simulink model "URController"  (R2023a)
settings: Solver=ode4  StartTime=0.0  StopTime=3  FixedStep=0.001  RelTol=1e-3  EnableMultiTasking=on
values from neighbouring files (symbols this model uses):
  CYCLE_FREQ = 0.001    [init.m]
  MAX_ACC = 100    [init.m]
  MAX_VEL = 180    [init.m]
libraries: slpidlib x13, forwardkinematics x2, simulink x1
(part 1 of 3)
settings Model: Creator=Steve  LastModifiedBy=Steve
settings SolverCC: AutoInsertRateTranBlk=on
settings DataIOCC: SaveOutput=off  SaveTime=off
settings OptimizationCC: DefaultParameterBehavior=Inlined  InlineInvariantSignals=on  EnhancedBackFolding=on  PassReuseOutputArgsAs=Individual arguments  StateBitsets=on  DataBitsets=on  ZeroExternalMemoryAtStartup=off  ZeroInternalMemoryAtStartup=off  NoFixptDivByZeroProtection=on  LifeSpan=1  OptimizeBlockOrder=speed  DifferentSizesBufferReuse=on  EfficientTunableParamExpr=on
settings DebuggingCC: ParameterTunabilityLossMsg=error  UnderSpecifiedDimensionMsg=warning
settings HardwareCC: ProdBitPerPointer=32  ProdBitPerSizeT=32  ProdBitPerPtrDiffT=32  ProdLargestAtomicFloat=None  ProdIntDivRoundTo=Floor  ProdWordSize=32  ProdHWDeviceType=Generic->Custom
settings SFSimCC: MATLABDynamicMemAlloc=off
settings RTWCC: Description=Embedded Coder  SystemTargetFile=ert.tlc  TLCOptions=-p0  GenCodeOnly=on  PackageGeneratedCodeAndArtifacts=on  TemplateMakefile=ert_default_tmf  GenerateReport=on  RTWVerbose=off  IncludeHyperlinkInReport=on  LaunchReport=on  TargetLang=C++
settings CodeAppCC: ForceParamTrailComments=on  IgnoreCustomStorageClasses=off  OperatorAnnotations=on  SimulinkDataObjDesc=on  SFDataObjDesc=on  CustomSymbolStrGlobalVar=rt$N$M  CustomSymbolStrType=$N$M  CustomSymbolStrFcn=$N$M$F  CustomSymbolStrMacro=$N$M  InsertBlockDesc=on
settings ERTTargetCC: TargetLangStandard=C++11 (ISO)  CodeReplacementLibrary=ISO_C  GenerateSampleERTMain=on  SupportAbsoluteTime=off  CodeInterfacePackaging=C++ class  SupportNonFinite=off  SupportComplex=off  SupportContinuousTime=on  SupportVariableSizeSignals=on  InlinedParameterPlacement=NonHierarchical  RootIOFormat=Structure reference  ERTDataSrcFileTemplate=data_h_template.cgt  ERTCustomFileTemplate=example_file_process.tlc

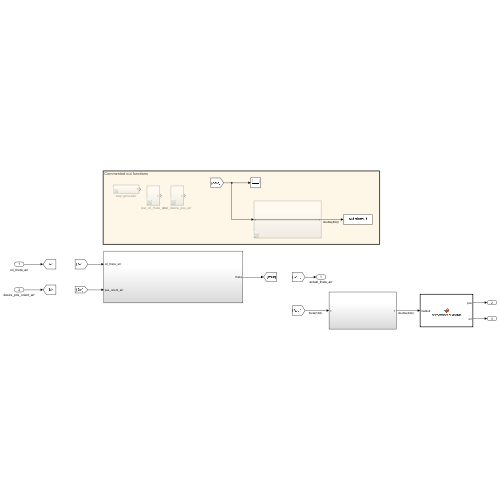
[thumbnail: Simulink's stored preview of the top-level diagram]
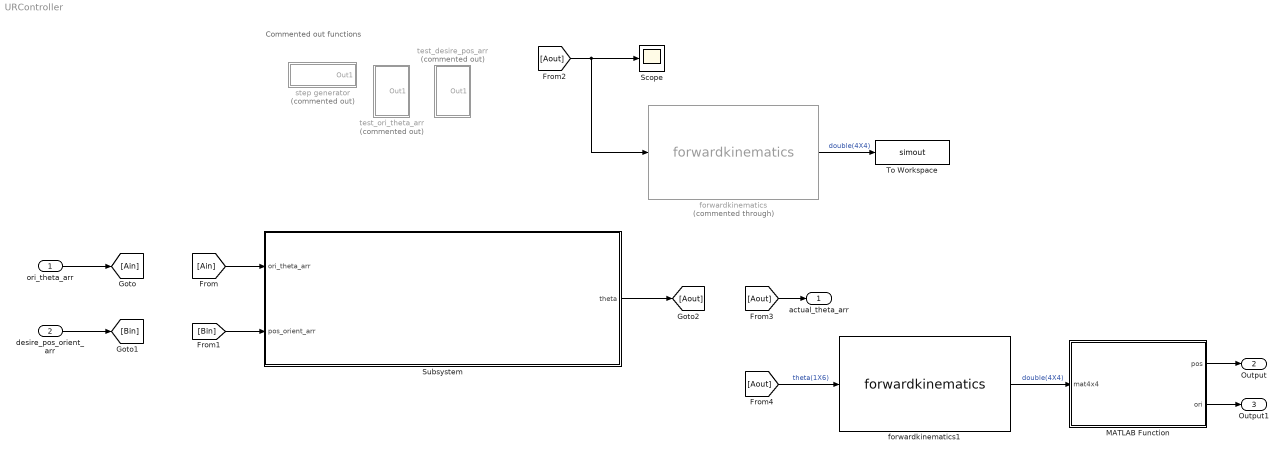
== system URController ==
  note: Commented out functions
  ori_theta_arr : Inport  OutDataTypeStr=double  PortDimensions=6
  desire_pos_orient_arr : Inport  Port=2  OutDataTypeStr=double  PortDimensions=6
  MATLAB Function : MATLAB Function  TreatAsAtomicUnit=on
  Scope : Scope
  Subsystem : Subsystem
  To Workspace : ToWorkspace  VariableName=simout  SaveFormat=Timeseries  SampleTime=-1
  forwardkinematics : forwardkinematics/forwardkinematics  Commented=through  SystemSampleTime=-1  VariantActivationTime=update diagram  Latency=0  AutoFrameSizeCalculation=off
      settings: SourceProductName=My Library
  forwardkinematics1 : forwardkinematics/forwardkinematics  SystemSampleTime=-1  VariantActivationTime=update diagram  Latency=0  AutoFrameSizeCalculation=off
      settings: SourceProductName=My Library
  step generator : Subsystem  Commented=on
  test_desire_pos_arr : Subsystem  Commented=on
  test_ori_theta_arr : Subsystem  Commented=on
  actual_theta_arr : Outport  OutDataTypeStr=double  PortDimensions=6
  Output : Outport  Port=2
  Output1 : Outport  Port=3
  wires:
  [Aout] -> Scope/1, forwardkinematics/1
  forwardkinematics/1 -> To Workspace/1  "double(4X4)"
  [Ain] -> Subsystem/1(ori_theta_arr)
  [Bin] -> Subsystem/2(pos_orient_arr)
  Subsystem/1(theta) -> [Aout]
  [Aout] -> actual_theta_arr/1
  [Aout] -> forwardkinematics1/1  "theta(1X6)"
  ori_theta_arr/1 -> [Ain]
  desire_pos_orient_arr/1 -> [Bin]
  forwardkinematics1/1 -> MATLAB Function/1(mat4x4)  "double(4X4)"
  MATLAB Function/1(pos) -> Output/1
  MATLAB Function/2(ori) -> Output1/1

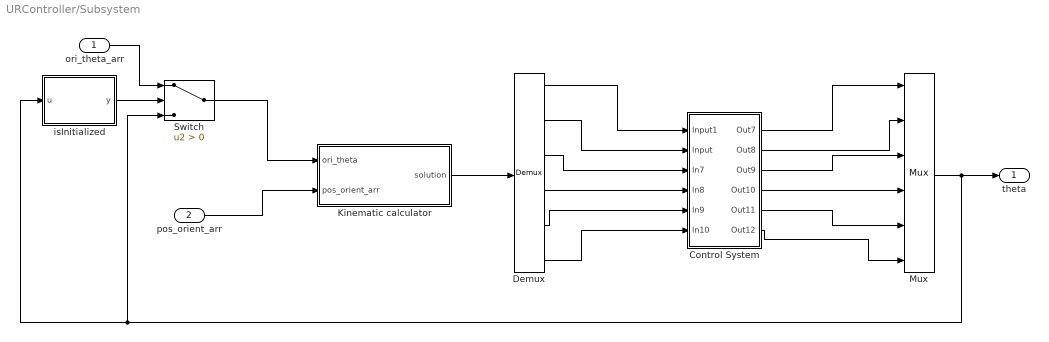
== system URController/Subsystem ==
  ori_theta_arr : Inport
  pos_orient_arr : Inport  Port=2
  Control System : Subsystem
  Demux : Demux  Outputs=6
  Kinematic calculator : Subsystem
  Mux : Mux  Inputs=6
  Switch : Switch  Criteria=u2 > Threshold  SaturateOnIntegerOverflow=off  InputSameDT=off
  isInitialized : MATLAB Function  TreatAsAtomicUnit=on
  theta : Outport
  wires:
  Mux/1 -> theta/1, isInitialized/1(u), Switch/3
  ori_theta_arr/1 -> Switch/1
  Switch/1 -> Kinematic calculator/1(ori_theta)
  Kinematic calculator/1(solution) -> Demux/1
  pos_orient_arr/1 -> Kinematic calculator/2(pos_orient_arr)
  isInitialized/1(y) -> Switch/2
  Demux/1 -> Control System/1(Input1)
  Demux/2 -> Control System/2(Input)
  Demux/3 -> Control System/3(In7)
  Demux/4 -> Control System/4(In8)
  Demux/5 -> Control System/5(In9)
  Demux/6 -> Control System/6(In10)
  Control System/1(Out7) -> Mux/1
  Control System/2(Out8) -> Mux/2
  Control System/3(Out9) -> Mux/3
  Control System/4(Out10) -> Mux/4
  Control System/5(Out11) -> Mux/5
  Control System/6(Out12) -> Mux/6

== system URController/step generator ==
  Clock : Clock
  Constant12 : Constant
  Constant13 : Constant  Value=[1 , 5 , 10 ,15]
  Floor : Rounding
  Selector : Selector  InputPortWidth=4  IndexOptions=Index vector (port)  Indices=[1 3]  OutputSizes=1
  Sum6 : Sum  Inputs=|++
  Out1 : Outport
  wires:
  Constant12/1 -> Sum6/2
  Constant13/1 -> Selector/1
  Selector/1 -> Out1/1
  Sum6/1 -> Floor/1
  Floor/1 -> Selector/2  "alpha"
  Clock/1 -> Sum6/1

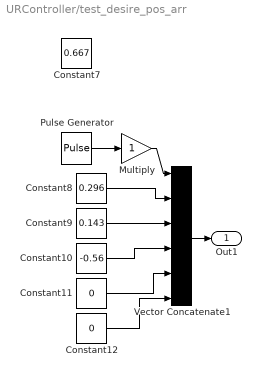
== system URController/test_desire_pos_arr ==
  Constant10 : Constant  Value=-0.56  OutDataTypeStr=double
  Constant11 : Constant  Value=0  OutDataTypeStr=double
  Constant12 : Constant  Value=0  OutDataTypeStr=double
  Constant7 : Constant  Value=0.667  OutDataTypeStr=double
  Constant8 : Constant  Value=0.296  OutDataTypeStr=double
  Constant9 : Constant  Value=0.143  OutDataTypeStr=double
  Multiply : Gain
  Pulse Generator : DiscretePulseGenerator  PulseType=Time based  Amplitude=0.01  Period=1  PulseWidth=20
  Vector Concatenate1 : Concatenate  NumInputs=6
  Out1 : Outport
  wires:
  Vector Concatenate1/1 -> Out1/1
  Constant12/1 -> Vector Concatenate1/6
  Constant11/1 -> Vector Concatenate1/5
  Constant9/1 -> Vector Concatenate1/3
  Constant10/1 -> Vector Concatenate1/4
  Pulse Generator/1 -> Multiply/1
  Constant8/1 -> Vector Concatenate1/2
  Multiply/1 -> Vector Concatenate1/1

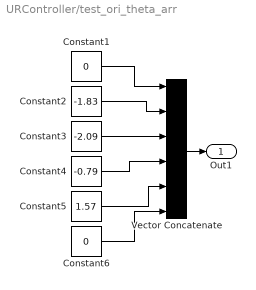
== system URController/test_ori_theta_arr ==
  Constant1 : Constant  Value=0  OutDataTypeStr=double
  Constant2 : Constant  Value=-1.83  OutDataTypeStr=double
  Constant3 : Constant  Value=-2.09  OutDataTypeStr=double
  Constant4 : Constant  Value=-0.79  OutDataTypeStr=double
  Constant5 : Constant  Value=1.57  OutDataTypeStr=double
  Constant6 : Constant  Value=0  OutDataTypeStr=double
  Vector Concatenate : Concatenate  NumInputs=6
  Out1 : Outport
  wires:
  Constant3/1 -> Vector Concatenate/3
  Constant4/1 -> Vector Concatenate/4
  Constant2/1 -> Vector Concatenate/2
  Constant1/1 -> Vector Concatenate/1
  Constant6/1 -> Vector Concatenate/6
  Constant5/1 -> Vector Concatenate/5
  Vector Concatenate/1 -> Out1/1

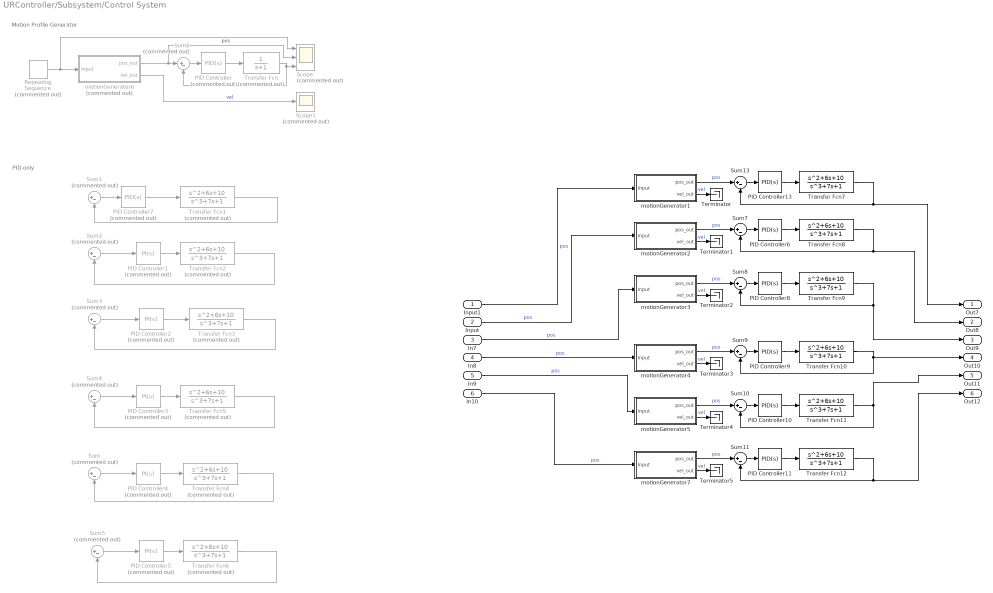
== system URController/Subsystem/Control System ==
  note: PID only
  note: Motion Profile Generator
  Input1 : Inport
  Input : Inport  Port=2
  In7 : Inport  Port=3
  In8 : Inport  Port=4
  In9 : Inport  Port=5
  In10 : Inport  Port=6
  PID Controller : slpidlib/PID Controller  Commented=on  Controller=PID  Form=Parallel  TimeDomain=Continuous-time  UseExternalTs=off  SampleTime=-1  IntegratorMethod=Forward Euler  FilterMethod=Forward Euler  ControllerParametersSource=internal  P=16.8294093394131  I=84.3967388731047  UseKiTs=off  D=-0.0900818829328251  N=186.823463181414  UseFilter=on  TunerSelectOption=Transfer Function Based (PID Tuner App)  InitialConditionSource=internal  InitialConditionForIntegrator=0  InitialConditionForFilter=0  DifferentiatorICPrevScaledInput=0  ExternalReset=none  TrackingMode=off  Kt=1  LimitOutput=off  SatLimitsSource=internal  UpperSaturationLimit=inf  LowerSaturationLimit=-inf  LinearizeAsGain=on  AntiWindupMode=none  Kb=1  LimitIntegrator=off  UpperIntegratorSaturationLimit=inf  LowerIntegratorSaturationLimit=-inf  POutMin=[]  POutMax=[]  IOutMin=[]  IOutMax=[]  DOutMin=[]  DOutMax=[]  NOutMin=[]  NOutMax=[]  SumOutMin=[]  SumOutMax=[]  SaturationOutMin=[]  SaturationOutMax=[]  PParamMin=[]  PParamMax=[]  IParamMin=[]  IParamMax=[]  DParamMin=[]  DParamMax=[]  NParamMin=[]  NParamMax=[]  KbParamMin=[]  KbParamMax=[]  KtParamMin=[]  KtParamMax=[]  KbOutMin=[]  KbOutMax=[]  KtOutMin=[]  KtOutMax=[]  IntegratorOutMin=[]  IntegratorOutMax=[]  FilterOutMin=[]  FilterOutMax=[]  SumI1OutMin=[]  SumI1OutMax=[]  SumI2OutMin=[]  SumI2OutMax=[]  SumI3OutMin=[]  SumI3OutMax=[]  SumI4OutMin=[]  SumI4OutMax=[]  SumDOutMin=[]  SumDOutMax=[]  DifferentiatorOutMin=[]  DifferentiatorOutMax=[]  FilterDiffOutCoefMin=[]  FilterDiffOutCoefMax=[]  ReciprocalOutMin=[]  ReciprocalOutMax=[]  SumDenOutMin=[]  SumDenOutMax=[]  SumNumOutMin=[]  SumNumOutMax=[]  DivideOutMin=[]  DivideOutMax=[]  UdiffTsProdOutMin=[]  UdiffTsProdOutMax=[]  NTsProdOutMin=[]  NTsProdOutMax=[]  UintegralTsProdOutMin=[]  UintegralTsProdOutMax=[]  UngainTsProdOutMin=[]  UngainTsProdOutMax=[]  ClampingZeroOutDataTypeStr=Inherit: Inherit via back propagation  ClampingZeroOutMin=[]  ClampingZeroOutMax=[]  FilterDenConstantOutDataTypeStr=Inherit: Inherit via back propagation  FilterDenConstantOutMin=[]  FilterDenConstantOutMax=[]  PCopyOutDataTypeStr=Inherit: Inherit via back propagation  PCopyOutMin=[]  PCopyOutMax=[]  NCopyOutDataTypeStr=Inherit: Inherit via back propagation  NCopyOutMin=[]  NCopyOutMax=[]  IntegratorContinuousStateAttributes=''  IntegratorStateMustResolveToSignalObject=off  IntegratorRTWStateStorageClass=Auto  FilterContinuousStateAttributes=''  FilterStateMustResolveToSignalObject=off  FilterRTWStateStorageClass=Auto  ParallelPVariant=InternalParameters  IdealPVariant=Disabled  IVariant=InternalParameters  DVariant=InternalParameters  IntegratorVariant=Continuous  SatVariant=Disabled  AWVariant=Passthrough  PCopyVariant=Disabled  TRVariant=Disabled  FdbkBlocksVariant=Forward  IdealPFdbkVariant=Disabled  SatFdbkVariant=Disabled  DerivativeFilterVariant=ContFilter  NVariant=InternalParameters  NCopyVariant=Disabled  FilterICVariant=InternalICsFilter  IntegratorICVariant=InternalICs  ExternalResetVariant=Disabled  TRSumVariant=Passthrough  SumFdbkVariant=Disabled  SumVariant=Sum_PID  TsampFilterVariant=InternalTs  TsampNgainVariant=Passthrough  TsampIntegralVariant=Disabled_SignalSpec  ExternalSaturationOutDataTypeStr=Inherit: Same as second input
  PID Controller1 : slpidlib/PID Controller  Commented=on  Controller=PI  Form=Parallel  TimeDomain=Continuous-time  UseExternalTs=off  SampleTime=-1  IntegratorMethod=Forward Euler  FilterMethod=Forward Euler  ControllerParametersSource=internal  P=107.100265619314  I=6616.60930018075  UseKiTs=off  D=-0.189486999754633  N=63.8304243098863  UseFilter=on  TunerSelectOption=Transfer Function Based (PID Tuner App)  InitialConditionSource=internal  InitialConditionForIntegrator=0  InitialConditionForFilter=0  DifferentiatorICPrevScaledInput=0  ExternalReset=none  TrackingMode=off  Kt=1  LimitOutput=off  SatLimitsSource=internal  UpperSaturationLimit=inf  LowerSaturationLimit=-inf  LinearizeAsGain=on  AntiWindupMode=none  Kb=1  LimitIntegrator=off  UpperIntegratorSaturationLimit=inf  LowerIntegratorSaturationLimit=-inf  POutMin=[]  POutMax=[]  IOutMin=[]  IOutMax=[]  DOutMin=[]  DOutMax=[]  NOutMin=[]  NOutMax=[]  SumOutMin=[]  SumOutMax=[]  SaturationOutMin=[]  SaturationOutMax=[]  PParamMin=[]  PParamMax=[]  IParamMin=[]  IParamMax=[]  DParamMin=[]  DParamMax=[]  NParamMin=[]  NParamMax=[]  KbParamMin=[]  KbParamMax=[]  KtParamMin=[]  KtParamMax=[]  KbOutMin=[]  KbOutMax=[]  KtOutMin=[]  KtOutMax=[]  IntegratorOutMin=[]  IntegratorOutMax=[]  FilterOutMin=[]  FilterOutMax=[]  SumI1OutMin=[]  SumI1OutMax=[]  SumI2OutMin=[]  SumI2OutMax=[]  SumI3OutMin=[]  SumI3OutMax=[]  SumI4OutMin=[]  SumI4OutMax=[]  SumDOutMin=[]  SumDOutMax=[]  DifferentiatorOutMin=[]  DifferentiatorOutMax=[]  FilterDiffOutCoefMin=[]  FilterDiffOutCoefMax=[]  ReciprocalOutMin=[]  ReciprocalOutMax=[]  SumDenOutMin=[]  SumDenOutMax=[]  SumNumOutMin=[]  SumNumOutMax=[]  DivideOutMin=[]  DivideOutMax=[]  UdiffTsProdOutMin=[]  UdiffTsProdOutMax=[]  NTsProdOutMin=[]  NTsProdOutMax=[]  UintegralTsProdOutMin=[]  UintegralTsProdOutMax=[]  UngainTsProdOutMin=[]  UngainTsProdOutMax=[]  ClampingZeroOutDataTypeStr=Inherit: Inherit via back propagation  ClampingZeroOutMin=[]  ClampingZeroOutMax=[]  FilterDenConstantOutDataTypeStr=Inherit: Inherit via back propagation  FilterDenConstantOutMin=[]  FilterDenConstantOutMax=[]  PCopyOutDataTypeStr=Inherit: Inherit via back propagation  PCopyOutMin=[]  PCopyOutMax=[]  NCopyOutDataTypeStr=Inherit: Inherit via back propagation  NCopyOutMin=[]  NCopyOutMax=[]  IntegratorContinuousStateAttributes=''  IntegratorStateMustResolveToSignalObject=off  IntegratorRTWStateStorageClass=Auto  FilterContinuousStateAttributes=''  FilterStateMustResolveToSignalObject=off  FilterRTWStateStorageClass=Auto  ParallelPVariant=InternalParameters  IdealPVariant=Disabled  IVariant=InternalParameters  DVariant=Disabled  IntegratorVariant=Continuous  SatVariant=Disabled  AWVariant=Passthrough  PCopyVariant=Disabled  TRVariant=Disabled  FdbkBlocksVariant=Forward  IdealPFdbkVariant=Disabled  SatFdbkVariant=Disabled  DerivativeFilterVariant=Disabled  NVariant=Disabled  NCopyVariant=Disabled_SignalSpec  FilterICVariant=Disabled  IntegratorICVariant=InternalICs  ExternalResetVariant=Disabled  TRSumVariant=Passthrough  SumFdbkVariant=Disabled  SumVariant=Sum_PI  TsampFilterVariant=InternalTs  TsampNgainVariant=Passthrough  TsampIntegralVariant=Disabled_SignalSpec  ExternalSaturationOutDataTypeStr=Inherit: Same as second input
  PID Controller{6,8..11,13} (6 alike) : slpidlib/PID Controller  Controller=PID  Form=Parallel  TimeDomain=Continuous-time  UseExternalTs=off  SampleTime=-1  IntegratorMethod=Forward Euler  FilterMethod=Forward Euler  ControllerParametersSource=internal  P=16.8294093394131  I=84.3967388731047  UseKiTs=off  D=-0.0900818829328251  N=186.823463181414  UseFilter=on  TunerSelectOption=Transfer Function Based (PID Tuner App)  InitialConditionSource=internal  InitialConditionForIntegrator=0  InitialConditionForFilter=0  DifferentiatorICPrevScaledInput=0  ExternalReset=none  TrackingMode=off  Kt=1  LimitOutput=off  SatLimitsSource=internal  UpperSaturationLimit=inf  LowerSaturationLimit=-inf  LinearizeAsGain=on  AntiWindupMode=none  Kb=1  LimitIntegrator=off  UpperIntegratorSaturationLimit=inf  LowerIntegratorSaturationLimit=-inf  POutMin=[]  POutMax=[]  IOutMin=[]  IOutMax=[]  DOutMin=[]  DOutMax=[]  NOutMin=[]  NOutMax=[]  SumOutMin=[]  SumOutMax=[]  SaturationOutMin=[]  SaturationOutMax=[]  PParamMin=[]  PParamMax=[]  IParamMin=[]  IParamMax=[]  DParamMin=[]  DParamMax=[]  NParamMin=[]  NParamMax=[]  KbParamMin=[]  KbParamMax=[]  KtParamMin=[]  KtParamMax=[]  KbOutMin=[]  KbOutMax=[]  KtOutMin=[]  KtOutMax=[]  IntegratorOutMin=[]  IntegratorOutMax=[]  FilterOutMin=[]  FilterOutMax=[]  SumI1OutMin=[]  SumI1OutMax=[]  SumI2OutMin=[]  SumI2OutMax=[]  SumI3OutMin=[]  SumI3OutMax=[]  SumI4OutMin=[]  SumI4OutMax=[]  SumDOutMin=[]  SumDOutMax=[]  DifferentiatorOutMin=[]  DifferentiatorOutMax=[]  FilterDiffOutCoefMin=[]  FilterDiffOutCoefMax=[]  ReciprocalOutMin=[]  ReciprocalOutMax=[]  SumDenOutMin=[]  SumDenOutMax=[]  SumNumOutMin=[]  SumNumOutMax=[]  DivideOutMin=[]  DivideOutMax=[]  UdiffTsProdOutMin=[]  UdiffTsProdOutMax=[]  NTsProdOutMin=[]  NTsProdOutMax=[]  UintegralTsProdOutMin=[]  UintegralTsProdOutMax=[]  UngainTsProdOutMin=[]  UngainTsProdOutMax=[]  ClampingZeroOutDataTypeStr=Inherit: Inherit via back propagation  ClampingZeroOutMin=[]  ClampingZeroOutMax=[]  FilterDenConstantOutDataTypeStr=Inherit: Inherit via back propagation  FilterDenConstantOutMin=[]  FilterDenConstantOutMax=[]  PCopyOutDataTypeStr=Inherit: Inherit via back propagation  PCopyOutMin=[]  PCopyOutMax=[]  NCopyOutDataTypeStr=Inherit: Inherit via back propagation  NCopyOutMin=[]  NCopyOutMax=[]  IntegratorContinuousStateAttributes=''  IntegratorStateMustResolveToSignalObject=off  IntegratorRTWStateStorageClass=Auto  FilterContinuousStateAttributes=''  FilterStateMustResolveToSignalObject=off  FilterRTWStateStorageClass=Auto  ParallelPVariant=InternalParameters  IdealPVariant=Disabled  IVariant=InternalParameters  DVariant=InternalParameters  IntegratorVariant=Continuous  SatVariant=Disabled  AWVariant=Passthrough  PCopyVariant=Disabled  TRVariant=Disabled  FdbkBlocksVariant=Forward  IdealPFdbkVariant=Disabled  SatFdbkVariant=Disabled  DerivativeFilterVariant=ContFilter  NVariant=InternalParameters  NCopyVariant=Disabled  FilterICVariant=InternalICsFilter  IntegratorICVariant=InternalICs  ExternalResetVariant=Disabled  TRSumVariant=Passthrough  SumFdbkVariant=Disabled  SumVariant=Sum_PID  TsampFilterVariant=InternalTs  TsampNgainVariant=Passthrough  TsampIntegralVariant=Disabled_SignalSpec  ExternalSaturationOutDataTypeStr=Inherit: Same as second input
  PID Controller2 : slpidlib/PID Controller  Commented=on  Controller=PI  Form=Parallel  TimeDomain=Continuous-time  UseExternalTs=off  SampleTime=-1  IntegratorMethod=Forward Euler  FilterMethod=Forward Euler  ControllerParametersSource=internal  P=107.100265619314  I=6616.60930018075  UseKiTs=off  D=-0.189486999754633  N=63.8304243098863  UseFilter=on  TunerSelectOption=Transfer Function Based (PID Tuner App)  InitialConditionSource=internal  InitialConditionForIntegrator=0  InitialConditionForFilter=0  DifferentiatorICPrevScaledInput=0  ExternalReset=none  TrackingMode=off  Kt=1  LimitOutput=off  SatLimitsSource=internal  UpperSaturationLimit=inf  LowerSaturationLimit=-inf  LinearizeAsGain=on  AntiWindupMode=none  Kb=1  LimitIntegrator=off  UpperIntegratorSaturationLimit=inf  LowerIntegratorSaturationLimit=-inf  POutMin=[]  POutMax=[]  IOutMin=[]  IOutMax=[]  DOutMin=[]  DOutMax=[]  NOutMin=[]  NOutMax=[]  SumOutMin=[]  SumOutMax=[]  SaturationOutMin=[]  SaturationOutMax=[]  PParamMin=[]  PParamMax=[]  IParamMin=[]  IParamMax=[]  DParamMin=[]  DParamMax=[]  NParamMin=[]  NParamMax=[]  KbParamMin=[]  KbParamMax=[]  KtParamMin=[]  KtParamMax=[]  KbOutMin=[]  KbOutMax=[]  KtOutMin=[]  KtOutMax=[]  IntegratorOutMin=[]  IntegratorOutMax=[]  FilterOutMin=[]  FilterOutMax=[]  SumI1OutMin=[]  SumI1OutMax=[]  SumI2OutMin=[]  SumI2OutMax=[]  SumI3OutMin=[]  SumI3OutMax=[]  SumI4OutMin=[]  SumI4OutMax=[]  SumDOutMin=[]  SumDOutMax=[]  DifferentiatorOutMin=[]  DifferentiatorOutMax=[]  FilterDiffOutCoefMin=[]  FilterDiffOutCoefMax=[]  ReciprocalOutMin=[]  ReciprocalOutMax=[]  SumDenOutMin=[]  SumDenOutMax=[]  SumNumOutMin=[]  SumNumOutMax=[]  DivideOutMin=[]  DivideOutMax=[]  UdiffTsProdOutMin=[]  UdiffTsProdOutMax=[]  NTsProdOutMin=[]  NTsProdOutMax=[]  UintegralTsProdOutMin=[]  UintegralTsProdOutMax=[]  UngainTsProdOutMin=[]  UngainTsProdOutMax=[]  ClampingZeroOutDataTypeStr=Inherit: Inherit via back propagation  ClampingZeroOutMin=[]  ClampingZeroOutMax=[]  FilterDenConstantOutDataTypeStr=Inherit: Inherit via back propagation  FilterDenConstantOutMin=[]  FilterDenConstantOutMax=[]  PCopyOutDataTypeStr=Inherit: Inherit via back propagation  PCopyOutMin=[]  PCopyOutMax=[]  NCopyOutDataTypeStr=Inherit: Inherit via back propagation  NCopyOutMin=[]  NCopyOutMax=[]  IntegratorContinuousStateAttributes=''  IntegratorStateMustResolveToSignalObject=off  IntegratorRTWStateStorageClass=Auto  FilterContinuousStateAttributes=''  FilterStateMustResolveToSignalObject=off  FilterRTWStateStorageClass=Auto  ParallelPVariant=InternalParameters  IdealPVariant=Disabled  IVariant=InternalParameters  DVariant=Disabled  IntegratorVariant=Continuous  SatVariant=Disabled  AWVariant=Passthrough  PCopyVariant=Disabled  TRVariant=Disabled  FdbkBlocksVariant=Forward  IdealPFdbkVariant=Disabled  SatFdbkVariant=Disabled  DerivativeFilterVariant=Disabled  NVariant=Disabled  NCopyVariant=Disabled_SignalSpec  FilterICVariant=Disabled  IntegratorICVariant=InternalICs  ExternalResetVariant=Disabled  TRSumVariant=Passthrough  SumFdbkVariant=Disabled  SumVariant=Sum_PI  TsampFilterVariant=InternalTs  TsampNgainVariant=Passthrough  TsampIntegralVariant=Disabled_SignalSpec  ExternalSaturationOutDataTypeStr=Inherit: Same as second input
  PID Controller3 : slpidlib/PID Controller  Commented=on  Controller=PI  Form=Parallel  TimeDomain=Continuous-time  UseExternalTs=off  SampleTime=-1  IntegratorMethod=Forward Euler  FilterMethod=Forward Euler  ControllerParametersSource=internal  P=107.100265619314  I=6616.60930018075  UseKiTs=off  D=-0.189486999754633  N=63.8304243098863  UseFilter=on  TunerSelectOption=Transfer Function Based (PID Tuner App)  InitialConditionSource=internal  InitialConditionForIntegrator=0  InitialConditionForFilter=0  DifferentiatorICPrevScaledInput=0  ExternalReset=none  TrackingMode=off  Kt=1  LimitOutput=off  SatLimitsSource=internal  UpperSaturationLimit=inf  LowerSaturationLimit=-inf  LinearizeAsGain=on  AntiWindupMode=none  Kb=1  LimitIntegrator=off  UpperIntegratorSaturationLimit=inf  LowerIntegratorSaturationLimit=-inf  POutMin=[]  POutMax=[]  IOutMin=[]  IOutMax=[]  DOutMin=[]  DOutMax=[]  NOutMin=[]  NOutMax=[]  SumOutMin=[]  SumOutMax=[]  SaturationOutMin=[]  SaturationOutMax=[]  PParamMin=[]  PParamMax=[]  IParamMin=[]  IParamMax=[]  DParamMin=[]  DParamMax=[]  NParamMin=[]  NParamMax=[]  KbParamMin=[]  KbParamMax=[]  KtParamMin=[]  KtParamMax=[]  KbOutMin=[]  KbOutMax=[]  KtOutMin=[]  KtOutMax=[]  IntegratorOutMin=[]  IntegratorOutMax=[]  FilterOutMin=[]  FilterOutMax=[]  SumI1OutMin=[]  SumI1OutMax=[]  SumI2OutMin=[]  SumI2OutMax=[]  SumI3OutMin=[]  SumI3OutMax=[]  SumI4OutMin=[]  SumI4OutMax=[]  SumDOutMin=[]  SumDOutMax=[]  DifferentiatorOutMin=[]  DifferentiatorOutMax=[]  FilterDiffOutCoefMin=[]  FilterDiffOutCoefMax=[]  ReciprocalOutMin=[]  ReciprocalOutMax=[]  SumDenOutMin=[]  SumDenOutMax=[]  SumNumOutMin=[]  SumNumOutMax=[]  DivideOutMin=[]  DivideOutMax=[]  UdiffTsProdOutMin=[]  UdiffTsProdOutMax=[]  NTsProdOutMin=[]  NTsProdOutMax=[]  UintegralTsProdOutMin=[]  UintegralTsProdOutMax=[]  UngainTsProdOutMin=[]  UngainTsProdOutMax=[]  ClampingZeroOutDataTypeStr=Inherit: Inherit via back propagation  ClampingZeroOutMin=[]  ClampingZeroOutMax=[]  FilterDenConstantOutDataTypeStr=Inherit: Inherit via back propagation  FilterDenConstantOutMin=[]  FilterDenConstantOutMax=[]  PCopyOutDataTypeStr=Inherit: Inherit via back propagation  PCopyOutMin=[]  PCopyOutMax=[]  NCopyOutDataTypeStr=Inherit: Inherit via back propagation  NCopyOutMin=[]  NCopyOutMax=[]  IntegratorContinuousStateAttributes=''  IntegratorStateMustResolveToSignalObject=off  IntegratorRTWStateStorageClass=Auto  FilterContinuousStateAttributes=''  FilterStateMustResolveToSignalObject=off  FilterRTWStateStorageClass=Auto  ParallelPVariant=InternalParameters  IdealPVariant=Disabled  IVariant=InternalParameters  DVariant=Disabled  IntegratorVariant=Continuous  SatVariant=Disabled  AWVariant=Passthrough  PCopyVariant=Disabled  TRVariant=Disabled  FdbkBlocksVariant=Forward  IdealPFdbkVariant=Disabled  SatFdbkVariant=Disabled  DerivativeFilterVariant=Disabled  NVariant=Disabled  NCopyVariant=Disabled_SignalSpec  FilterICVariant=Disabled  IntegratorICVariant=InternalICs  ExternalResetVariant=Disabled  TRSumVariant=Passthrough  SumFdbkVariant=Disabled  SumVariant=Sum_PI  TsampFilterVariant=InternalTs  TsampNgainVariant=Passthrough  TsampIntegralVariant=Disabled_SignalSpec  ExternalSaturationOutDataTypeStr=Inherit: Same as second input
  PID Controller4 : slpidlib/PID Controller  Commented=on  Controller=PI  Form=Parallel  TimeDomain=Continuous-time  UseExternalTs=off  SampleTime=-1  IntegratorMethod=Forward Euler  FilterMethod=Forward Euler  ControllerParametersSource=internal  P=107.100265619314  I=6616.60930018075  UseKiTs=off  D=0  N=100  UseFilter=on  TunerSelectOption=Transfer Function Based (PID Tuner App)  InitialConditionSource=internal  InitialConditionForIntegrator=0  InitialConditionForFilter=0  DifferentiatorICPrevScaledInput=0  ExternalReset=none  TrackingMode=off  Kt=1  LimitOutput=off  SatLimitsSource=internal  UpperSaturationLimit=inf  LowerSaturationLimit=-inf  LinearizeAsGain=on  AntiWindupMode=none  Kb=1  LimitIntegrator=off  UpperIntegratorSaturationLimit=inf  LowerIntegratorSaturationLimit=-inf  POutMin=[]  POutMax=[]  IOutMin=[]  IOutMax=[]  DOutMin=[]  DOutMax=[]  NOutMin=[]  NOutMax=[]  SumOutMin=[]  SumOutMax=[]  SaturationOutMin=[]  SaturationOutMax=[]  PParamMin=[]  PParamMax=[]  IParamMin=[]  IParamMax=[]  DParamMin=[]  DParamMax=[]  NParamMin=[]  NParamMax=[]  KbParamMin=[]  KbParamMax=[]  KtParamMin=[]  KtParamMax=[]  KbOutMin=[]  KbOutMax=[]  KtOutMin=[]  KtOutMax=[]  IntegratorOutMin=[]  IntegratorOutMax=[]  FilterOutMin=[]  FilterOutMax=[]  SumI1OutMin=[]  SumI1OutMax=[]  SumI2OutMin=[]  SumI2OutMax=[]  SumI3OutMin=[]  SumI3OutMax=[]  SumI4OutMin=[]  SumI4OutMax=[]  SumDOutMin=[]  SumDOutMax=[]  DifferentiatorOutMin=[]  DifferentiatorOutMax=[]  FilterDiffOutCoefMin=[]  FilterDiffOutCoefMax=[]  ReciprocalOutMin=[]  ReciprocalOutMax=[]  SumDenOutMin=[]  SumDenOutMax=[]  SumNumOutMin=[]  SumNumOutMax=[]  DivideOutMin=[]  DivideOutMax=[]  UdiffTsProdOutMin=[]  UdiffTsProdOutMax=[]  NTsProdOutMin=[]  NTsProdOutMax=[]  UintegralTsProdOutMin=[]  UintegralTsProdOutMax=[]  UngainTsProdOutMin=[]  UngainTsProdOutMax=[]  ClampingZeroOutDataTypeStr=Inherit: Inherit via back propagation  ClampingZeroOutMin=[]  ClampingZeroOutMax=[]  FilterDenConstantOutDataTypeStr=Inherit: Inherit via back propagation  FilterDenConstantOutMin=[]  FilterDenConstantOutMax=[]  PCopyOutDataTypeStr=Inherit: Inherit via back propagation  PCopyOutMin=[]  PCopyOutMax=[]  NCopyOutDataTypeStr=Inherit: Inherit via back propagation  NCopyOutMin=[]  NCopyOutMax=[]  IntegratorContinuousStateAttributes=''  IntegratorStateMustResolveToSignalObject=off  IntegratorRTWStateStorageClass=Auto  FilterContinuousStateAttributes=''  FilterStateMustResolveToSignalObject=off  FilterRTWStateStorageClass=Auto  ParallelPVariant=InternalParameters  IdealPVariant=Disabled  IVariant=InternalParameters  DVariant=Disabled  IntegratorVariant=Continuous  SatVariant=Disabled  AWVariant=Passthrough  PCopyVariant=Disabled  TRVariant=Disabled  FdbkBlocksVariant=Forward  IdealPFdbkVariant=Disabled  SatFdbkVariant=Disabled  DerivativeFilterVariant=Disabled  NVariant=Disabled  NCopyVariant=Disabled_SignalSpec  FilterICVariant=Disabled  IntegratorICVariant=InternalICs  ExternalResetVariant=Disabled  TRSumVariant=Passthrough  SumFdbkVariant=Disabled  SumVariant=Sum_PI  TsampFilterVariant=InternalTs  TsampNgainVariant=Passthrough  TsampIntegralVariant=Disabled_SignalSpec  ExternalSaturationOutDataTypeStr=Inherit: Same as second input
  PID Controller5 : slpidlib/PID Controller  Commented=on  Controller=PI  Form=Parallel  TimeDomain=Continuous-time  UseExternalTs=off  SampleTime=-1  IntegratorMethod=Forward Euler  FilterMethod=Forward Euler  ControllerParametersSource=internal  P=107.100265619314  I=6616.60930018075  UseKiTs=off  D=0  N=100  UseFilter=on  TunerSelectOption=Transfer Function Based (PID Tuner App)  InitialConditionSource=internal  InitialConditionForIntegrator=0  InitialConditionForFilter=0  DifferentiatorICPrevScaledInput=0  ExternalReset=none  TrackingMode=off  Kt=1  LimitOutput=off  SatLimitsSource=internal  UpperSaturationLimit=inf  LowerSaturationLimit=-inf  LinearizeAsGain=on  AntiWindupMode=none  Kb=1  LimitIntegrator=off  UpperIntegratorSaturationLimit=inf  LowerIntegratorSaturationLimit=-inf  POutMin=[]  POutMax=[]  IOutMin=[]  IOutMax=[]  DOutMin=[]  DOutMax=[]  NOutMin=[]  NOutMax=[]  SumOutMin=[]  SumOutMax=[]  SaturationOutMin=[]  SaturationOutMax=[]  PParamMin=[]  PParamMax=[]  IParamMin=[]  IParamMax=[]  DParamMin=[]  DParamMax=[]  NParamMin=[]  NParamMax=[]  KbParamMin=[]  KbParamMax=[]  KtParamMin=[]  KtParamMax=[]  KbOutMin=[]  KbOutMax=[]  KtOutMin=[]  KtOutMax=[]  IntegratorOutMin=[]  IntegratorOutMax=[]  FilterOutMin=[]  FilterOutMax=[]  SumI1OutMin=[]  SumI1OutMax=[]  SumI2OutMin=[]  SumI2OutMax=[]  SumI3OutMin=[]  SumI3OutMax=[]  SumI4OutMin=[]  SumI4OutMax=[]  SumDOutMin=[]  SumDOutMax=[]  DifferentiatorOutMin=[]  DifferentiatorOutMax=[]  FilterDiffOutCoefMin=[]  FilterDiffOutCoefMax=[]  ReciprocalOutMin=[]  ReciprocalOutMax=[]  SumDenOutMin=[]  SumDenOutMax=[]  SumNumOutMin=[]  SumNumOutMax=[]  DivideOutMin=[]  DivideOutMax=[]  UdiffTsProdOutMin=[]  UdiffTsProdOutMax=[]  NTsProdOutMin=[]  NTsProdOutMax=[]  UintegralTsProdOutMin=[]  UintegralTsProdOutMax=[]  UngainTsProdOutMin=[]  UngainTsProdOutMax=[]  ClampingZeroOutDataTypeStr=Inherit: Inherit via back propagation  ClampingZeroOutMin=[]  ClampingZeroOutMax=[]  FilterDenConstantOutDataTypeStr=Inherit: Inherit via back propagation  FilterDenConstantOutMin=[]  FilterDenConstantOutMax=[]  PCopyOutDataTypeStr=Inherit: Inherit via back propagation  PCopyOutMin=[]  PCopyOutMax=[]  NCopyOutDataTypeStr=Inherit: Inherit via back propagation  NCopyOutMin=[]  NCopyOutMax=[]  IntegratorContinuousStateAttributes=''  IntegratorStateMustResolveToSignalObject=off  IntegratorRTWStateStorageClass=Auto  FilterContinuousStateAttributes=''  FilterStateMustResolveToSignalObject=off  FilterRTWStateStorageClass=Auto  ParallelPVariant=InternalParameters  IdealPVariant=Disabled  IVariant=InternalParameters  DVariant=Disabled  IntegratorVariant=Continuous  SatVariant=Disabled  AWVariant=Passthrough  PCopyVariant=Disabled  TRVariant=Disabled  FdbkBlocksVariant=Forward  IdealPFdbkVariant=Disabled  SatFdbkVariant=Disabled  DerivativeFilterVariant=Disabled  NVariant=Disabled  NCopyVariant=Disabled_SignalSpec  FilterICVariant=Disabled  IntegratorICVariant=InternalICs  ExternalResetVariant=Disabled  TRSumVariant=Passthrough  SumFdbkVariant=Disabled  SumVariant=Sum_PI  TsampFilterVariant=InternalTs  TsampNgainVariant=Passthrough  TsampIntegralVariant=Disabled_SignalSpec  ExternalSaturationOutDataTypeStr=Inherit: Same as second input
  PID Controller7 : slpidlib/PID Controller  Commented=on  Controller=PID  Form=Parallel  TimeDomain=Continuous-time  UseExternalTs=off  SampleTime=-1  IntegratorMethod=Forward Euler  FilterMethod=Forward Euler  ControllerParametersSource=internal  P=47.3438798562812  I=206.276392279903  UseKiTs=off  D=-0.189486999754633  N=63.8304243098863  UseFilter=on  TunerSelectOption=Transfer Function Based (PID Tuner App)  InitialConditionSource=internal  InitialConditionForIntegrator=0  InitialConditionForFilter=0  DifferentiatorICPrevScaledInput=0  ExternalReset=none  TrackingMode=off  Kt=1  LimitOutput=off  SatLimitsSource=internal  UpperSaturationLimit=inf  LowerSaturationLimit=-inf  LinearizeAsGain=on  AntiWindupMode=none  Kb=1  LimitIntegrator=off  UpperIntegratorSaturationLimit=inf  LowerIntegratorSaturationLimit=-inf  POutMin=[]  POutMax=[]  IOutMin=[]  IOutMax=[]  DOutMin=[]  DOutMax=[]  NOutMin=[]  NOutMax=[]  SumOutMin=[]  SumOutMax=[]  SaturationOutMin=[]  SaturationOutMax=[]  PParamMin=[]  PParamMax=[]  IParamMin=[]  IParamMax=[]  DParamMin=[]  DParamMax=[]  NParamMin=[]  NParamMax=[]  KbParamMin=[]  KbParamMax=[]  KtParamMin=[]  KtParamMax=[]  KbOutMin=[]  KbOutMax=[]  KtOutMin=[]  KtOutMax=[]  IntegratorOutMin=[]  IntegratorOutMax=[]  FilterOutMin=[]  FilterOutMax=[]  SumI1OutMin=[]  SumI1OutMax=[]  SumI2OutMin=[]  SumI2OutMax=[]  SumI3OutMin=[]  SumI3OutMax=[]  SumI4OutMin=[]  SumI4OutMax=[]  SumDOutMin=[]  SumDOutMax=[]  DifferentiatorOutMin=[]  DifferentiatorOutMax=[]  FilterDiffOutCoefMin=[]  FilterDiffOutCoefMax=[]  ReciprocalOutMin=[]  ReciprocalOutMax=[]  SumDenOutMin=[]  SumDenOutMax=[]  SumNumOutMin=[]  SumNumOutMax=[]  DivideOutMin=[]  DivideOutMax=[]  UdiffTsProdOutMin=[]  UdiffTsProdOutMax=[]  NTsProdOutMin=[]  NTsProdOutMax=[]  UintegralTsProdOutMin=[]  UintegralTsProdOutMax=[]  UngainTsProdOutMin=[]  UngainTsProdOutMax=[]  ClampingZeroOutDataTypeStr=Inherit: Inherit via back propagation  ClampingZeroOutMin=[]  ClampingZeroOutMax=[]  FilterDenConstantOutDataTypeStr=Inherit: Inherit via back propagation  FilterDenConstantOutMin=[]  FilterDenConstantOutMax=[]  PCopyOutDataTypeStr=Inherit: Inherit via back propagation  PCopyOutMin=[]  PCopyOutMax=[]  NCopyOutDataTypeStr=Inherit: Inherit via back propagation  NCopyOutMin=[]  NCopyOutMax=[]  IntegratorContinuousStateAttributes=''  IntegratorStateMustResolveToSignalObject=off  IntegratorRTWStateStorageClass=Auto  FilterContinuousStateAttributes=''  FilterStateMustResolveToSignalObject=off  FilterRTWStateStorageClass=Auto  ParallelPVariant=InternalParameters  IdealPVariant=Disabled  IVariant=InternalParameters  DVariant=InternalParameters  IntegratorVariant=Continuous  SatVariant=Disabled  AWVariant=Passthrough  PCopyVariant=Disabled  TRVariant=Disabled  FdbkBlocksVariant=Forward  IdealPFdbkVariant=Disabled  SatFdbkVariant=Disabled  DerivativeFilterVariant=ContFilter  NVariant=InternalParameters  NCopyVariant=Disabled  FilterICVariant=InternalICsFilter  IntegratorICVariant=InternalICs  ExternalResetVariant=Disabled  TRSumVariant=Passthrough  SumFdbkVariant=Disabled  SumVariant=Sum_PID  TsampFilterVariant=InternalTs  TsampNgainVariant=Passthrough  TsampIntegralVariant=Disabled_SignalSpec  ExternalSaturationOutDataTypeStr=Inherit: Same as second input
  Repeating Sequence : simulink/Sources/Repeating Sequence  Commented=on  rep_seq_t="[0    0.1    0.5   0.6    1    1.1   2    2.1    3]"  rep_seq_y="[0     1      1       2    2      3   3       4      4]"
  Scope : Scope  Commented=on  NumInputPorts=3
  Scope1 : Scope  Commented=on
  Sum{,1..6} (7 alike) : Sum  Commented=on  Inputs=|+-
  Sum{7..11,13} (6 alike) : Sum  Inputs=|+-
  Terminator{,1..5} (6 alike) : Terminator
  Transfer Fcn : TransferFcn  Commented=on  Denominator=[1 1]
  Transfer Fcn{1..6} (6 alike) : TransferFcn  Commented=on  Numerator=[1 6 10]  Denominator=[1 0 7 1]
  Transfer Fcn{7..12} (6 alike) : TransferFcn  Numerator=[1 6 10]  Denominator=[1 0 7 1]
  motionGenerator1 : Subsystem
  motionGenerator2 : Subsystem
  motionGenerator3 : Subsystem
  motionGenerator4 : Subsystem
  motionGenerator5 : Subsystem
  motionGenerator6 : Subsystem  Commented=on
  motionGenerator7 : Subsystem
  Out7 : Outport
  Out8 : Outport  Port=2
  Out9 : Outport  Port=3
  Out10 : Outport  Port=4
  Out11 : Outport  Port=5
  Out12 : Outport  Port=6
  wires:
  Transfer Fcn2/1 -> Sum2/2
  Transfer Fcn4/1 -> Sum/2
  Sum3/1 -> PID Controller2/1
  Transfer Fcn3/1 -> Sum3/2
  PID Controller1/1 -> Transfer Fcn2/1
  PID Controller5/1 -> Transfer Fcn6/1
  Transfer Fcn5/1 -> Sum4/2
  Sum5/1 -> PID Controller5/1
  PID Controller4/1 -> Transfer Fcn4/1
  PID Controller3/1 -> Transfer Fcn5/1
  Sum2/1 -> PID Controller1/1
  Transfer Fcn6/1 -> Sum5/2
  Sum4/1 -> PID Controller3/1
  Sum/1 -> PID Controller4/1
  PID Controller2/1 -> Transfer Fcn3/1
  PID Controller7/1 -> Transfer Fcn1/1
  Transfer Fcn1/1 -> Sum1/2
  Sum1/1 -> PID Controller7/1
  motionGenerator6/2(vel_out) -> Scope1/1  "vel"
  Transfer Fcn/1 -> Scope/3, Sum6/2
  PID Controller/1 -> Transfer Fcn/1
  Sum6/1 -> PID Controller/1
  motionGenerator6/1(pos_out) -> Scope/2, Sum6/1  "pos"
  Repeating Sequence/1 -> motionGenerator6/1(Input), Scope/1
  Input1/1 -> motionGenerator1/1(Input)  "pos"
  PID Controller13/1 -> Transfer Fcn7/1
  Transfer Fcn7/1 -> Sum13/2, Out7/1
  Sum13/1 -> PID Controller13/1
  motionGenerator1/1(pos_out) -> Sum13/1  "pos"
  motionGenerator1/2(vel_out) -> Terminator/1  "vel"
  motionGenerator2/2(vel_out) -> Terminator1/1  "vel"
  Sum7/1 -> PID Controller6/1
  PID Controller6/1 -> Transfer Fcn8/1
  motionGenerator2/1(pos_out) -> Sum7/1  "pos"
  Transfer Fcn8/1 -> Out8/1, Sum7/2
  Input/1 -> motionGenerator2/1(Input)  "pos"
  motionGenerator3/2(vel_out) -> Terminator2/1  "vel"
  Sum8/1 -> PID Controller8/1
  PID Controller8/1 -> Transfer Fcn9/1
  motionGenerator3/1(pos_out) -> Sum8/1  "pos"
  Transfer Fcn9/1 -> Out9/1, Sum8/2
  In7/1 -> motionGenerator3/1(Input)  "pos"
  motionGenerator4/2(vel_out) -> Terminator3/1  "vel"
  Sum9/1 -> PID Controller9/1
  PID Controller9/1 -> Transfer Fcn10/1
  motionGenerator4/1(pos_out) -> Sum9/1  "pos"
  Transfer Fcn10/1 -> Sum9/2, Out10/1
  In8/1 -> motionGenerator4/1(Input)  "pos"
  motionGenerator5/2(vel_out) -> Terminator4/1  "vel"
  Sum10/1 -> PID Controller10/1
  PID Controller10/1 -> Transfer Fcn11/1
  motionGenerator5/1(pos_out) -> Sum10/1  "pos"
  Transfer Fcn11/1 -> Sum10/2, Out11/1
  In9/1 -> motionGenerator5/1(Input)  "pos"
  motionGenerator7/2(vel_out) -> Terminator5/1  "vel"
  Sum11/1 -> PID Controller11/1
  PID Controller11/1 -> Transfer Fcn12/1
  motionGenerator7/1(pos_out) -> Sum11/1  "pos"
  Transfer Fcn12/1 -> Out12/1, Sum11/2
  In10/1 -> motionGenerator7/1(Input)  "pos"

== system URController/Subsystem/Kinematic calculator ==
  ori_theta : Inport
  pos_orient_arr : Inport  Port=2
  MATLAB Function : MATLAB Function  TreatAsAtomicUnit=on
  MATLAB Function1 : MATLAB Function  TreatAsAtomicUnit=on
  MATLAB Function2 : MATLAB Function  TreatAsAtomicUnit=on
  solution : Outport
  wires:
  MATLAB Function1/1(gd) -> MATLAB Function/1(gd)
  MATLAB Function/1(theta) -> MATLAB Function2/2(theta)
  MATLAB Function2/1(solution) -> solution/1
  pos_orient_arr/1 -> MATLAB Function1/1(pos_orient_arr)
  ori_theta/1 -> MATLAB Function2/1(ori_theta)

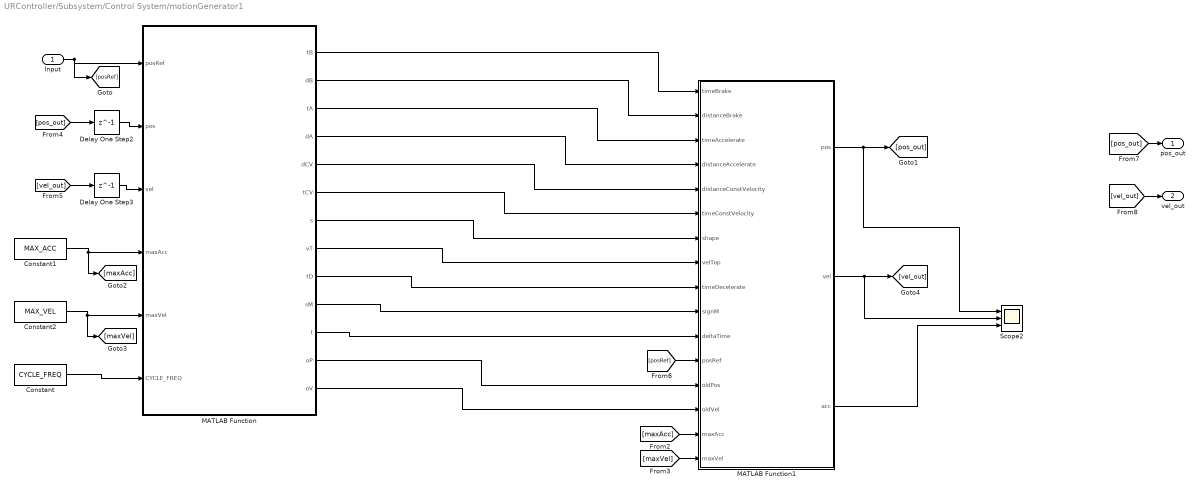
== system URController/Subsystem/Control System/motionGenerator1 ==
  Input : Inport
  Constant : Constant  Value=CYCLE_FREQ
  Constant1 : Constant  Value=MAX_ACC
  Constant2 : Constant  Value=MAX_VEL
  Delay One Step2 : Delay  DelayLength=1
  Delay One Step3 : Delay  DelayLength=1
  MATLAB Function : MATLAB Function  TreatAsAtomicUnit=on
  MATLAB Function1 : MATLAB Function  TreatAsAtomicUnit=on
  Scope2 : Scope  NumInputPorts=3
  pos_out : Outport
  vel_out : Outport  Port=2
  wires:
  [vel_out] -> Delay One Step3/1
  Delay One Step3/1 -> MATLAB Function/3(vel)
  MATLAB Function/9(tD) -> MATLAB Function1/9(timeDecelerate)
  Constant2/1 -> [maxVel], MATLAB Function/5(maxVel)
  MATLAB Function/5(dCV) -> MATLAB Function1/5(distanceConstVelocity)
  [pos_out] -> Delay One Step2/1
  MATLAB Function/8(vT) -> MATLAB Function1/8(velTop)
  MATLAB Function/2(dB) -> MATLAB Function1/2(distanceBrake)
  MATLAB Function1/2(vel) -> Scope2/2, [vel_out]
  Constant1/1 -> [maxAcc], MATLAB Function/4(maxAcc)
  [maxAcc] -> MATLAB Function1/15(maxAcc)
  MATLAB Function/1(tB) -> MATLAB Function1/1(timeBrake)
  MATLAB Function1/1(pos) -> Scope2/1, [pos_out]
  MATLAB Function/11(t) -> MATLAB Function1/11(deltaTime)
  Delay One Step2/1 -> MATLAB Function/2(pos)
  MATLAB Function/7(s) -> MATLAB Function1/7(shape)
  MATLAB Function/10(sM) -> MATLAB Function1/10(signM)
  MATLAB Function/6(tCV) -> MATLAB Function1/6(timeConstVelocity)
  Input/1 -> [posRef], MATLAB Function/1(posRef)
  [maxVel] -> MATLAB Function1/16(maxVel)
  MATLAB Function/4(dA) -> MATLAB Function1/4(distanceAccelerate)
  MATLAB Function/3(tA) -> MATLAB Function1/3(timeAccelerate)
  [posRef] -> MATLAB Function1/12(posRef)
  MATLAB Function1/3(acc) -> Scope2/3
  [pos_out] -> pos_out/1
  [vel_out] -> vel_out/1
  Constant/1 -> MATLAB Function/6(CYCLE_FREQ)
  MATLAB Function/12(oP) -> MATLAB Function1/13(oldPos)
  MATLAB Function/13(oV) -> MATLAB Function1/14(oldVel)

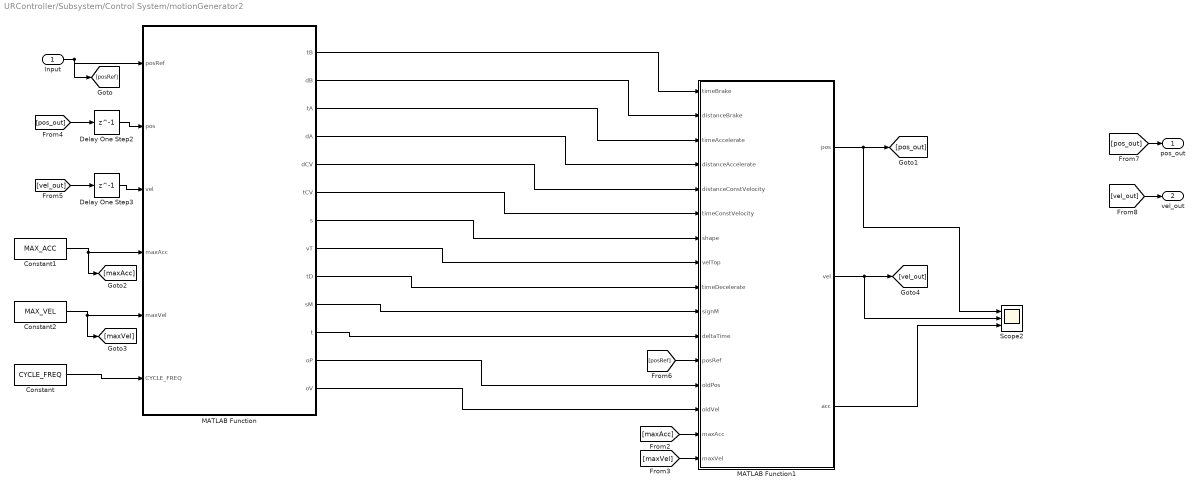
== system URController/Subsystem/Control System/motionGenerator2 ==
  Input : Inport
  Constant : Constant  Value=CYCLE_FREQ
  Constant1 : Constant  Value=MAX_ACC
  Constant2 : Constant  Value=MAX_VEL
  Delay One Step2 : Delay  DelayLength=1
  Delay One Step3 : Delay  DelayLength=1
  MATLAB Function : MATLAB Function  TreatAsAtomicUnit=on
  MATLAB Function1 : MATLAB Function  TreatAsAtomicUnit=on
  Scope2 : Scope  NumInputPorts=3
  pos_out : Outport
  vel_out : Outport  Port=2
  wires:
  [vel_out] -> Delay One Step3/1
  Delay One Step3/1 -> MATLAB Function/3(vel)
  MATLAB Function/9(tD) -> MATLAB Function1/9(timeDecelerate)
  Constant2/1 -> [maxVel], MATLAB Function/5(maxVel)
  MATLAB Function/5(dCV) -> MATLAB Function1/5(distanceConstVelocity)
  [pos_out] -> Delay One Step2/1
  MATLAB Function/8(vT) -> MATLAB Function1/8(velTop)
  MATLAB Function/2(dB) -> MATLAB Function1/2(distanceBrake)
  MATLAB Function1/2(vel) -> Scope2/2, [vel_out]
  Constant1/1 -> [maxAcc], MATLAB Function/4(maxAcc)
  [maxAcc] -> MATLAB Function1/15(maxAcc)
  MATLAB Function/1(tB) -> MATLAB Function1/1(timeBrake)
  MATLAB Function1/1(pos) -> Scope2/1, [pos_out]
  MATLAB Function/11(t) -> MATLAB Function1/11(deltaTime)
  Delay One Step2/1 -> MATLAB Function/2(pos)
  MATLAB Function/7(s) -> MATLAB Function1/7(shape)
  MATLAB Function/10(sM) -> MATLAB Function1/10(signM)
  MATLAB Function/6(tCV) -> MATLAB Function1/6(timeConstVelocity)
  Input/1 -> [posRef], MATLAB Function/1(posRef)
  [maxVel] -> MATLAB Function1/16(maxVel)
  MATLAB Function/4(dA) -> MATLAB Function1/4(distanceAccelerate)
  MATLAB Function/3(tA) -> MATLAB Function1/3(timeAccelerate)
  [posRef] -> MATLAB Function1/12(posRef)
  MATLAB Function1/3(acc) -> Scope2/3
  [pos_out] -> pos_out/1
  [vel_out] -> vel_out/1
  Constant/1 -> MATLAB Function/6(CYCLE_FREQ)
  MATLAB Function/12(oP) -> MATLAB Function1/13(oldPos)
  MATLAB Function/13(oV) -> MATLAB Function1/14(oldVel)

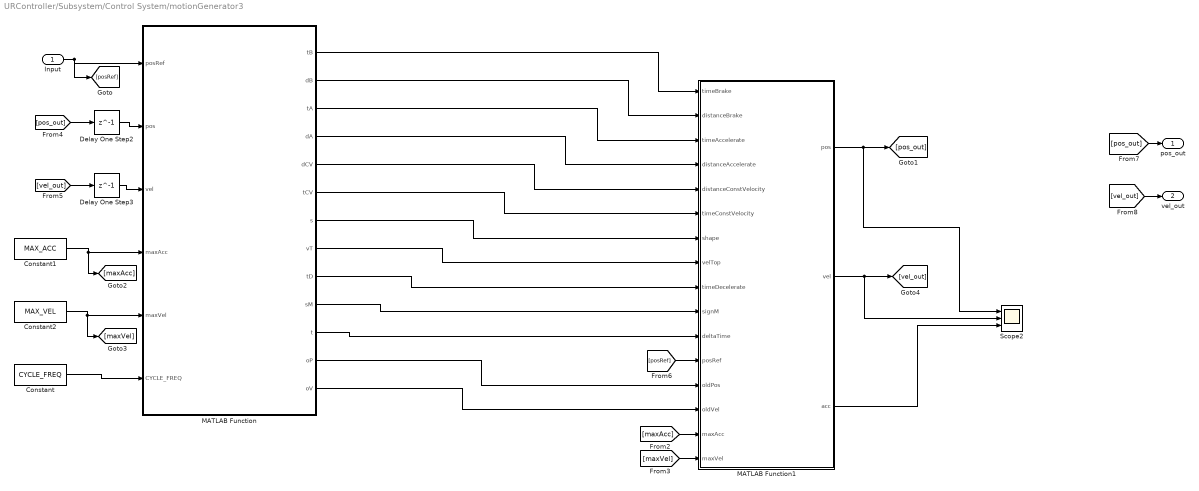
== system URController/Subsystem/Control System/motionGenerator3 ==
  Input : Inport
  Constant : Constant  Value=CYCLE_FREQ
  Constant1 : Constant  Value=MAX_ACC
  Constant2 : Constant  Value=MAX_VEL
  Delay One Step2 : Delay  DelayLength=1
  Delay One Step3 : Delay  DelayLength=1
  MATLAB Function : MATLAB Function  TreatAsAtomicUnit=on
  MATLAB Function1 : MATLAB Function  TreatAsAtomicUnit=on
  Scope2 : Scope  NumInputPorts=3
  pos_out : Outport
  vel_out : Outport  Port=2
  wires:
  [vel_out] -> Delay One Step3/1
  Delay One Step3/1 -> MATLAB Function/3(vel)
  MATLAB Function/9(tD) -> MATLAB Function1/9(timeDecelerate)
  Constant2/1 -> [maxVel], MATLAB Function/5(maxVel)
  MATLAB Function/5(dCV) -> MATLAB Function1/5(distanceConstVelocity)
  [pos_out] -> Delay One Step2/1
  MATLAB Function/8(vT) -> MATLAB Function1/8(velTop)
  MATLAB Function/2(dB) -> MATLAB Function1/2(distanceBrake)
  MATLAB Function1/2(vel) -> Scope2/2, [vel_out]
  Constant1/1 -> [maxAcc], MATLAB Function/4(maxAcc)
  [maxAcc] -> MATLAB Function1/15(maxAcc)
  MATLAB Function/1(tB) -> MATLAB Function1/1(timeBrake)
  MATLAB Function1/1(pos) -> Scope2/1, [pos_out]
  MATLAB Function/11(t) -> MATLAB Function1/11(deltaTime)
  Delay One Step2/1 -> MATLAB Function/2(pos)
  MATLAB Function/7(s) -> MATLAB Function1/7(shape)
  MATLAB Function/10(sM) -> MATLAB Function1/10(signM)
  MATLAB Function/6(tCV) -> MATLAB Function1/6(timeConstVelocity)
  Input/1 -> [posRef], MATLAB Function/1(posRef)
  [maxVel] -> MATLAB Function1/16(maxVel)
  MATLAB Function/4(dA) -> MATLAB Function1/4(distanceAccelerate)
  MATLAB Function/3(tA) -> MATLAB Function1/3(timeAccelerate)
  [posRef] -> MATLAB Function1/12(posRef)
  MATLAB Function1/3(acc) -> Scope2/3
  [pos_out] -> pos_out/1
  [vel_out] -> vel_out/1
  Constant/1 -> MATLAB Function/6(CYCLE_FREQ)
  MATLAB Function/12(oP) -> MATLAB Function1/13(oldPos)
  MATLAB Function/13(oV) -> MATLAB Function1/14(oldVel)

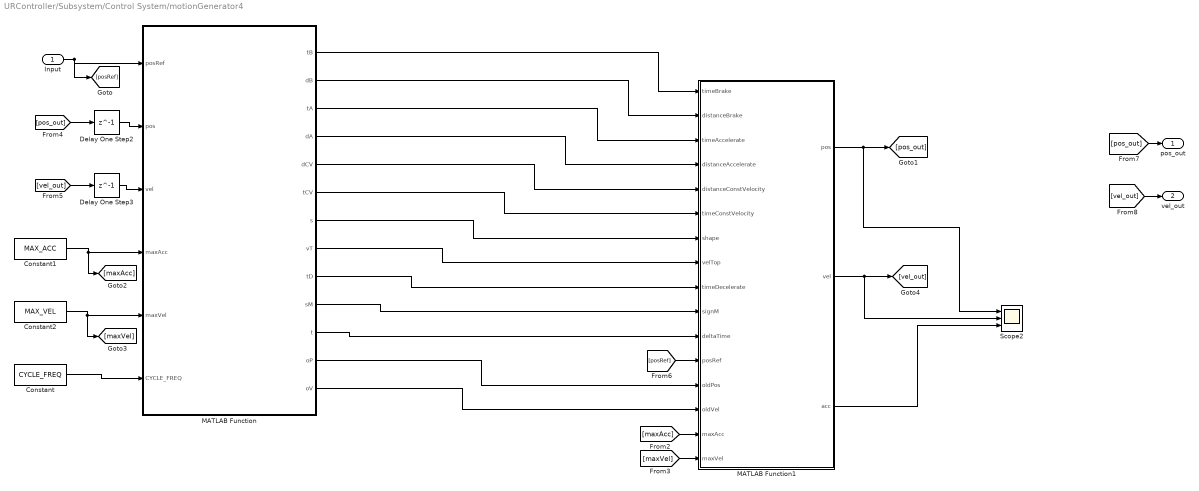
== system URController/Subsystem/Control System/motionGenerator4 ==
  Input : Inport
  Constant : Constant  Value=CYCLE_FREQ
  Constant1 : Constant  Value=MAX_ACC
  Constant2 : Constant  Value=MAX_VEL
  Delay One Step2 : Delay  DelayLength=1
  Delay One Step3 : Delay  DelayLength=1
  MATLAB Function : MATLAB Function  TreatAsAtomicUnit=on
  MATLAB Function1 : MATLAB Function  TreatAsAtomicUnit=on
  Scope2 : Scope  NumInputPorts=3
  pos_out : Outport
  vel_out : Outport  Port=2
  wires:
  [vel_out] -> Delay One Step3/1
  Delay One Step3/1 -> MATLAB Function/3(vel)
  MATLAB Function/9(tD) -> MATLAB Function1/9(timeDecelerate)
  Constant2/1 -> [maxVel], MATLAB Function/5(maxVel)
  MATLAB Function/5(dCV) -> MATLAB Function1/5(distanceConstVelocity)
  [pos_out] -> Delay One Step2/1
  MATLAB Function/8(vT) -> MATLAB Function1/8(velTop)
  MATLAB Function/2(dB) -> MATLAB Function1/2(distanceBrake)
  MATLAB Function1/2(vel) -> Scope2/2, [vel_out]
  Constant1/1 -> [maxAcc], MATLAB Function/4(maxAcc)
  [maxAcc] -> MATLAB Function1/15(maxAcc)
  MATLAB Function/1(tB) -> MATLAB Function1/1(timeBrake)
  MATLAB Function1/1(pos) -> Scope2/1, [pos_out]
  MATLAB Function/11(t) -> MATLAB Function1/11(deltaTime)
  Delay One Step2/1 -> MATLAB Function/2(pos)
  MATLAB Function/7(s) -> MATLAB Function1/7(shape)
  MATLAB Function/10(sM) -> MATLAB Function1/10(signM)
  MATLAB Function/6(tCV) -> MATLAB Function1/6(timeConstVelocity)
  Input/1 -> [posRef], MATLAB Function/1(posRef)
  [maxVel] -> MATLAB Function1/16(maxVel)
  MATLAB Function/4(dA) -> MATLAB Function1/4(distanceAccelerate)
  MATLAB Function/3(tA) -> MATLAB Function1/3(timeAccelerate)
  [posRef] -> MATLAB Function1/12(posRef)
  MATLAB Function1/3(acc) -> Scope2/3
  [pos_out] -> pos_out/1
  [vel_out] -> vel_out/1
  Constant/1 -> MATLAB Function/6(CYCLE_FREQ)
  MATLAB Function/12(oP) -> MATLAB Function1/13(oldPos)
  MATLAB Function/13(oV) -> MATLAB Function1/14(oldVel)

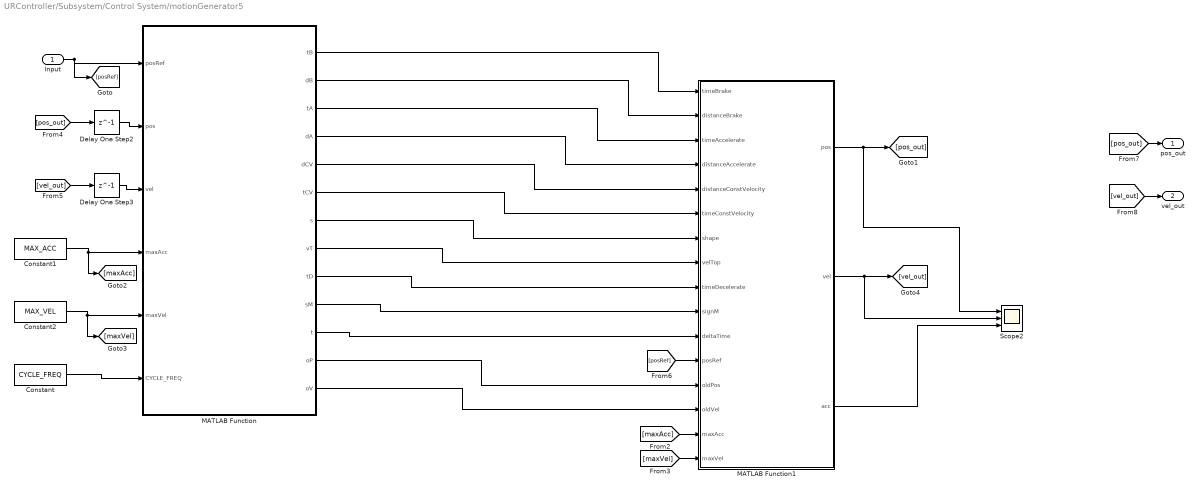
== system URController/Subsystem/Control System/motionGenerator5 ==
  Input : Inport
  Constant : Constant  Value=CYCLE_FREQ
  Constant1 : Constant  Value=MAX_ACC
  Constant2 : Constant  Value=MAX_VEL
  Delay One Step2 : Delay  DelayLength=1
  Delay One Step3 : Delay  DelayLength=1
  MATLAB Function : MATLAB Function  TreatAsAtomicUnit=on
  MATLAB Function1 : MATLAB Function  TreatAsAtomicUnit=on
  Scope2 : Scope  NumInputPorts=3
  pos_out : Outport
  vel_out : Outport  Port=2
  wires:
  [vel_out] -> Delay One Step3/1
  Delay One Step3/1 -> MATLAB Function/3(vel)
  MATLAB Function/9(tD) -> MATLAB Function1/9(timeDecelerate)
  Constant2/1 -> [maxVel], MATLAB Function/5(maxVel)
  MATLAB Function/5(dCV) -> MATLAB Function1/5(distanceConstVelocity)
  [pos_out] -> Delay One Step2/1
  MATLAB Function/8(vT) -> MATLAB Function1/8(velTop)
  MATLAB Function/2(dB) -> MATLAB Function1/2(distanceBrake)
  MATLAB Function1/2(vel) -> Scope2/2, [vel_out]
  Constant1/1 -> [maxAcc], MATLAB Function/4(maxAcc)
  [maxAcc] -> MATLAB Function1/15(maxAcc)
  MATLAB Function/1(tB) -> MATLAB Function1/1(timeBrake)
  MATLAB Function1/1(pos) -> Scope2/1, [pos_out]
  MATLAB Function/11(t) -> MATLAB Function1/11(deltaTime)
  Delay One Step2/1 -> MATLAB Function/2(pos)
  MATLAB Function/7(s) -> MATLAB Function1/7(shape)
  MATLAB Function/10(sM) -> MATLAB Function1/10(signM)
  MATLAB Function/6(tCV) -> MATLAB Function1/6(timeConstVelocity)
  Input/1 -> [posRef], MATLAB Function/1(posRef)
  [maxVel] -> MATLAB Function1/16(maxVel)
  MATLAB Function/4(dA) -> MATLAB Function1/4(distanceAccelerate)
  MATLAB Function/3(tA) -> MATLAB Function1/3(timeAccelerate)
  [posRef] -> MATLAB Function1/12(posRef)
  MATLAB Function1/3(acc) -> Scope2/3
  [pos_out] -> pos_out/1
  [vel_out] -> vel_out/1
  Constant/1 -> MATLAB Function/6(CYCLE_FREQ)
  MATLAB Function/12(oP) -> MATLAB Function1/13(oldPos)
  MATLAB Function/13(oV) -> MATLAB Function1/14(oldVel)

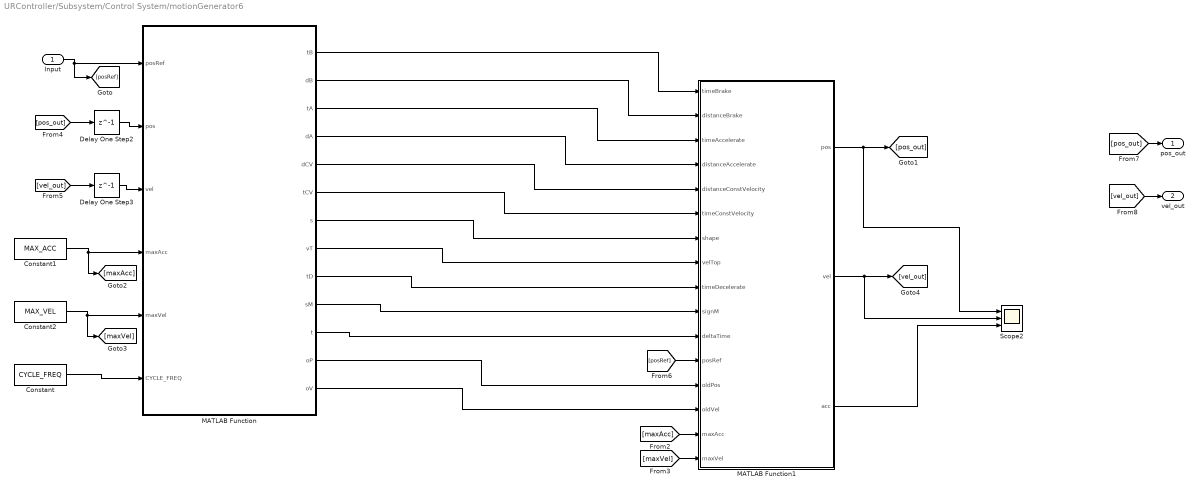
== system URController/Subsystem/Control System/motionGenerator6 ==
  Input : Inport
  Constant : Constant  Value=CYCLE_FREQ
  Constant1 : Constant  Value=MAX_ACC
  Constant2 : Constant  Value=MAX_VEL
  Delay One Step2 : Delay  DelayLength=1
  Delay One Step3 : Delay  DelayLength=1
  MATLAB Function : MATLAB Function  TreatAsAtomicUnit=on
  MATLAB Function1 : MATLAB Function  TreatAsAtomicUnit=on
  Scope2 : Scope  NumInputPorts=3
  pos_out : Outport
  vel_out : Outport  Port=2
  wires:
  [vel_out] -> Delay One Step3/1
  Delay One Step3/1 -> MATLAB Function/3(vel)
  MATLAB Function/9(tD) -> MATLAB Function1/9(timeDecelerate)
  Constant2/1 -> [maxVel], MATLAB Function/5(maxVel)
  MATLAB Function/5(dCV) -> MATLAB Function1/5(distanceConstVelocity)
  [pos_out] -> Delay One Step2/1
  MATLAB Function/8(vT) -> MATLAB Function1/8(velTop)
  MATLAB Function/2(dB) -> MATLAB Function1/2(distanceBrake)
  MATLAB Function1/2(vel) -> Scope2/2, [vel_out]
  Constant1/1 -> [maxAcc], MATLAB Function/4(maxAcc)
  [maxAcc] -> MATLAB Function1/15(maxAcc)
  MATLAB Function/1(tB) -> MATLAB Function1/1(timeBrake)
  MATLAB Function1/1(pos) -> Scope2/1, [pos_out]
  MATLAB Function/11(t) -> MATLAB Function1/11(deltaTime)
  Delay One Step2/1 -> MATLAB Function/2(pos)
  MATLAB Function/7(s) -> MATLAB Function1/7(shape)
  MATLAB Function/10(sM) -> MATLAB Function1/10(signM)
  MATLAB Function/6(tCV) -> MATLAB Function1/6(timeConstVelocity)
  Input/1 -> [posRef], MATLAB Function/1(posRef)
  [maxVel] -> MATLAB Function1/16(maxVel)
  MATLAB Function/4(dA) -> MATLAB Function1/4(distanceAccelerate)
  MATLAB Function/3(tA) -> MATLAB Function1/3(timeAccelerate)
  [posRef] -> MATLAB Function1/12(posRef)
  MATLAB Function1/3(acc) -> Scope2/3
  [pos_out] -> pos_out/1
  [vel_out] -> vel_out/1
  Constant/1 -> MATLAB Function/6(CYCLE_FREQ)
  MATLAB Function/12(oP) -> MATLAB Function1/13(oldPos)
  MATLAB Function/13(oV) -> MATLAB Function1/14(oldVel)
